simulink model "Lidar"  (R2022b)
settings: Solver=FixedStepAuto  StartTime=0.0  StopTime=10  FixedStep=Ts  RelTol=1e-3
InitFcn:
  | Ts=0.01;
model workspace (MAT data in the model file):
  SL_ROS_VariableLengthArrays_MaxSizes.CommonInfo.ArrayTruncateAction = 'EmitWarning'
  SL_ROS_VariableLengthArrays_MaxSizes.MsgTypeMap = containers.Map
  SL_ROS_VariableLengthArrays_MaxSizes.MsgTypeMap.serialization.keys = {'sensor_msgs/LaserScan', 'std_msgs/Header'}
  SL_ROS_VariableLengthArrays_MaxSizes.MsgTypeMap.serialization.values{1}(1).PropertyName = 'intensities'
  SL_ROS_VariableLengthArrays_MaxSizes.MsgTypeMap.serialization.values{1}(1).DataType = 'single'
  SL_ROS_VariableLengthArrays_MaxSizes.MsgTypeMap.serialization.values{1}(1).MaxLength = 1
  SL_ROS_VariableLengthArrays_MaxSizes.MsgTypeMap.serialization.values{1}(2).PropertyName = 'ranges'
  SL_ROS_VariableLengthArrays_MaxSizes.MsgTypeMap.serialization.values{1}(2).DataType = 'single'
  SL_ROS_VariableLengthArrays_MaxSizes.MsgTypeMap.serialization.values{1}(2).MaxLength = 6
  SL_ROS_VariableLengthArrays_MaxSizes.MsgTypeMap.serialization.values{2}.PropertyName = 'frame_id'
  SL_ROS_VariableLengthArrays_MaxSizes.MsgTypeMap.serialization.values{2}.DataType = 'uint8'
  SL_ROS_VariableLengthArrays_MaxSizes.MsgTypeMap.serialization.values{2}.MaxLength = 11
  SL_ROS_VariableLengthArrays_MaxSizes.MsgTypeMap.serialization.uniformity = 0
  SL_ROS_VariableLengthArrays_MaxSizes.MsgTypeMap.serialization.keyType = 'char'
  SL_ROS_VariableLengthArrays_MaxSizes.MsgTypeMap.serialization.valueType = 'any'
undefined symbols (not defined in the file): angle_increment, angle_max, angle_min, AngleFSA, AngleLSA, diffAngle, header, intensities, lidar_frame, range_max, range_min, ranges
libraries: ros2lib x3, simulink_extras x3, instrumentseriallib x2
settings Model: Creator=System-10  LastModifiedBy=System-10
settings DataIOCC: ExternalInput=AngleFSA
settings OptimizationCC: EnhancedBackFolding=on  PassReuseOutputArgsAs=Individual arguments  ZeroExternalMemoryAtStartup=off  ZeroInternalMemoryAtStartup=off  MaxStackSize=64  OptimizeBlockOrder=speed  DifferentSizesBufferReuse=on  OptimizationCustomize=off  EfficientTunableParamExpr=on
settings DebuggingCC: ParameterTunabilityLossMsg=error
settings HardwareCC: TargetBitPerPointer=64  TargetBitPerSizeT=64  TargetBitPerPtrDiffT=64  TargetLargestAtomicFloat=Float  TargetIntDivRoundTo=Zero  TargetEndianess=LittleEndian  TargetWordSize=64  TargetHWDeviceType=Intel->x86-64 (Windows64)
settings ModelReferenceCC: PropagateVarSize=During execution
settings SFSimCC: SimTargetLang=C++
settings RTWCC: Description=Embedded Coder  SystemTargetFile=ert.tlc  HardwareBoard=Robot Operating System 2 (ROS 2)  TLCOptions="-aInlineSetEventsForThisBaseRateFcn=TLC_FALSE -aSuppressMultiTaskScheduler=TLC_FALSE  -aRateBasedStepFcn=0"  TemplateMakefile=ert_default_tmf  Toolchain=Colcon Tools  TargetLang=C++
settings CodeAppCC: ForceParamTrailComments=on  IgnoreCustomStorageClasses=off  OperatorAnnotations=on  SimulinkDataObjDesc=on  SFDataObjDesc=on  InsertBlockDesc=on
settings ERTTargetCC: CodeInterfacePackaging=C++ class  SupportVariableSizeSignals=on  RootIOFormat=Structure reference

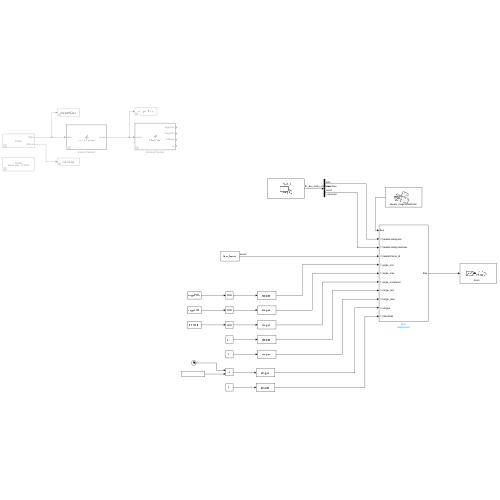
[thumbnail: Simulink's stored preview of the top-level diagram]
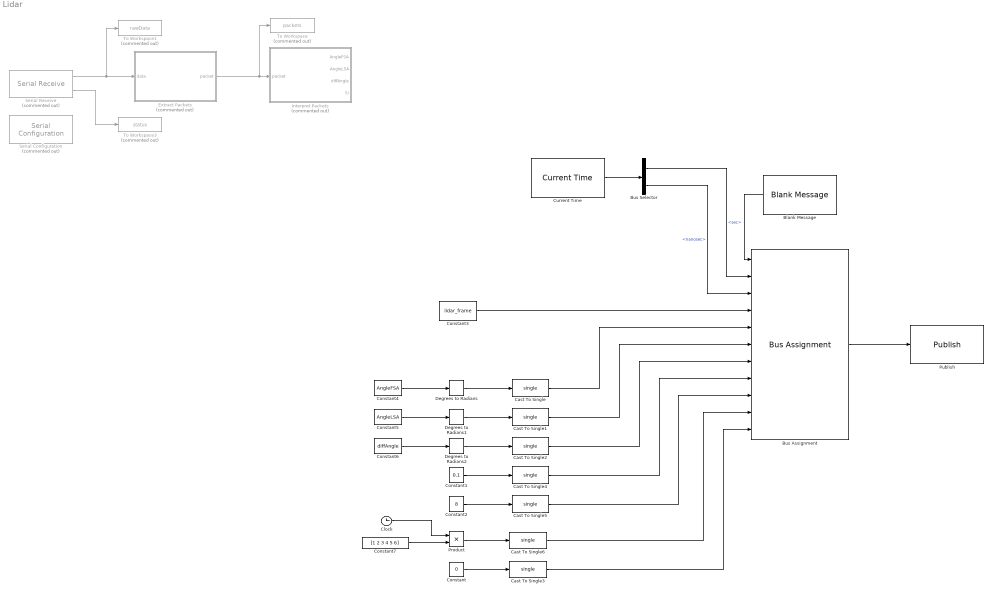
== system Lidar ==
  Blank Message : ros2lib/Blank Message  messageClass=Message  entityType=sensor_msgs/LaserScan  messageType=sensor_msgs/LaserScan  SampleTime=Ts
      settings: LibrarySourceBlock=roslib/ROS 2/Blank Message
  Bus Assignment : BusAssignment  AssignedSignals=header.stamp.sec,header.stamp.nanosec,header.frame_id,angle_min,angle_max,angle_increment,range_min,range_max,ranges,intensities
  Bus Selector : BusSelector  OutputSignals=sec,nanosec
  Cast To Single{,1..6} (7 alike) : DataTypeConversion  OutDataTypeStr=single  SaturateOnIntegerOverflow=off  RndMeth=Floor
  Clock : Clock
  Constant : Constant  Value=0
  Constant1 : Constant  Value=0.1
  Constant2 : Constant  Value=8
  Constant3 : Constant  Value=lidar_frame  VectorParams1D=off  OutDataTypeStr=uint8
  Constant4 : Constant  Value=AngleFSA
  Constant5 : Constant  Value=AngleLSA
  Constant6 : Constant  Value=diffAngle
  Constant7 : Constant  Value=[1 2 3 4 5 6]
  Current Time : ros2lib/Current Time  OutputFormat=bus  SampleTime=-1  ModelName=Lidar
      settings: LibrarySourceBlock=roslib/ROS 2/Current Time
  Degrees to Radians : simulink_extras/Transformations/Degrees to Radians
  Degrees to Radians1 : simulink_extras/Transformations/Degrees to Radians
  Degrees to Radians2 : simulink_extras/Transformations/Degrees to Radians
  Extract Packets : MATLAB Function  Commented=on  TreatAsAtomicUnit=on
  Interpret Packets : MATLAB Function  Commented=on  TreatAsAtomicUnit=on
  Product : Product
  Publish : ros2lib/Publish  topicSource=Specify your own  topic=/scan  messageType=sensor_msgs/LaserScan  QOSHistory=Keep last  QOSDepth=1  QOSReliability=Reliable  QOSDurability=Volatile
      settings: LibrarySourceBlock=roslib/ROS 2/Publish
  Serial Configuration : instrumentseriallib/Serial Configuration  Priority=-200000  Commented=on  PortSel=COM9  Port=COM9  ComPort=COM9  BaudRate=115200  DataBits=8  Parity=none  StopBits=1  ByteOrder=little-endian  FlowControl=none  Timeout=10  SimulateUsing=Interpreted execution  BlockInModel=on  aMode=1
  Serial Receive : instrumentseriallib/Serial Receive  Priority=1  Commented=on  PortSel=COM9  Port=COM9  ComPort=COM9  DataType=uint8  SaveDataType=uint8  ToggleHeader=off  Header=[170 85]  ToggleTerminator=off  Terminator=<none>  CustomTerminator=[]  InputFormat=Column major  ToggleDataSize=on  DataSize=[1 2000]  EnableBlockingMode=off  ActionDataUnavailable=Output last received value  ActionWhenDataUnavailable=Output last received value  CustomValue=111  SampleTime=Ts  SimulateUsing=Interpreted execution  BlockInModel=on  aMode=1
  To Workspace : ToWorkspace  Commented=on  VariableName=packets  SaveFormat=Timeseries  SampleTime=-1
  To Workspace1 : ToWorkspace  Commented=on  VariableName=rawData  SaveFormat=Structure  SampleTime=-1
      settings: Save2DSignal=2-D array (concatenate along first dimension)
  To Workspace3 : ToWorkspace  Commented=on  VariableName=status  SaveFormat=Structure  SampleTime=-1
      settings: Save2DSignal=2-D array (concatenate along first dimension)
  wires:
  Serial Receive/1 -> To Workspace1/1, Extract Packets/1(data)
  Serial Receive/2 -> To Workspace3/1
  Extract Packets/1(packet) -> Interpret Packets/1(packet), To Workspace/1
  Blank Message/1 -> Bus Assignment/1
  Cast To Single/1 -> Bus Assignment/5
  Cast To Single1/1 -> Bus Assignment/6
  Cast To Single2/1 -> Bus Assignment/7
  Constant/1 -> Cast To Single3/1
  Cast To Single3/1 -> Bus Assignment/11
  Cast To Single4/1 -> Bus Assignment/8
  Cast To Single5/1 -> Bus Assignment/9
  Constant1/1 -> Cast To Single4/1
  Constant2/1 -> Cast To Single5/1
  Cast To Single6/1 -> Bus Assignment/10
  Current Time/1 -> Bus Selector/1
  Bus Selector/1 -> Bus Assignment/2  "<sec>"
  Bus Selector/2 -> Bus Assignment/3  "<nanosec>"
  Bus Assignment/1 -> Publish/1
  Constant5/1 -> Degrees to Radians1/1
  Constant4/1 -> Degrees to Radians/1
  Constant6/1 -> Degrees to Radians2/1
  Constant7/1 -> Product/2
  Clock/1 -> Product/1
  Product/1 -> Cast To Single6/1
  Degrees to Radians2/1 -> Cast To Single2/1
  Degrees to Radians1/1 -> Cast To Single1/1
  Degrees to Radians/1 -> Cast To Single/1
  Constant3/1 -> Bus Assignment/4

== matlab function Lidar/Extract Packets ==
  data: data input; packet output double size=[100 100]
function packet = extractPackets(data)
    persistent indicesOfHeaders;
    persistent startIdx;
    persistent endIdx;
    persistent idx;
    persistent lastData;

    if isempty(lastData)
        lastData = uint8(zeros(1,size(data,2)));
    end

    if isempty(indicesOfHeaders) || ~isequal(data, lastData)
        
        indicesOfAA = find(data == 170);
        indicesOfHeaders = zeros(1, length(indicesOfAA)); 
        count = 0;
        
        startIdx = 0;
        endIdx = 0;
        idx = 0;

        for i = 1:length(indicesOfAA)
            if indicesOfAA(i) < length(data) && data(indicesOfAA(i) + 1) == 85
                count = count + 1;
                indicesOfHeaders(count) = indicesOfAA(i);
            end
        end

        indicesOfHeaders = indicesOfHeaders(1:count);
        lastData = data;      
    end
    
    if endIdx < indicesOfHeaders(end)
        idx = idx + 1;
        startIdx = indicesOfHeaders(idx);
        endIdx = indicesOfHeaders(idx+1);
        packet = double(data(startIdx:endIdx-1));
    else
        packet = [];
    end
end

== matlab function Lidar/Interpret Packets ==
  settings: sampleTime=0.01
  data: packet input; AngleFSA output; AngleLSA output; diffAngle output; Si output
function [AngleFSA, AngleLSA, diffAngle, Si] = interpreter(packet)

    AngleFSA = 0;
    AngleLSA = 0;
    diffAngle = 0;
    Si = zeros(1, 40);

    if size(packet, 2) < 90
        return;
    end

    FSA = double(bitor(bitshift(uint16(packet(1, 6)), 8), uint16(packet(1, 5)), 'uint16'));
    LSA = double(bitor(bitshift(uint16(packet(1, 8)), 8), uint16(packet(1, 7)), 'uint16'));
   
    AngleFSA = double(bitshift(FSA, -1) / 64);
    AngleLSA = double(bitshift(LSA, -1) / 64);
    diffAngle = mod((AngleLSA - AngleFSA),360);
    
    rawSi = uint8(packet(:, 11:end));

    for i = 1:2:length(rawSi)
        Si((i + 1) / 2) = double(bitor(bitshift(uint16(rawSi(1, i + 1)), 8), uint16(rawSi(1, i)), 'uint16'));
    end
    Si = Si / 4000;
end
